simulink model "RIN251129_16_18_L2"  (R2016b)
settings: Solver=VariableStepAuto  StartTime=0.0  StopTime=0.01  RelTol=1e-3
libraries: powerlib x31, powerlib_meascontrol x13
settings Model: Creator=ADMINISTRATOR  LastModifiedBy=Victor

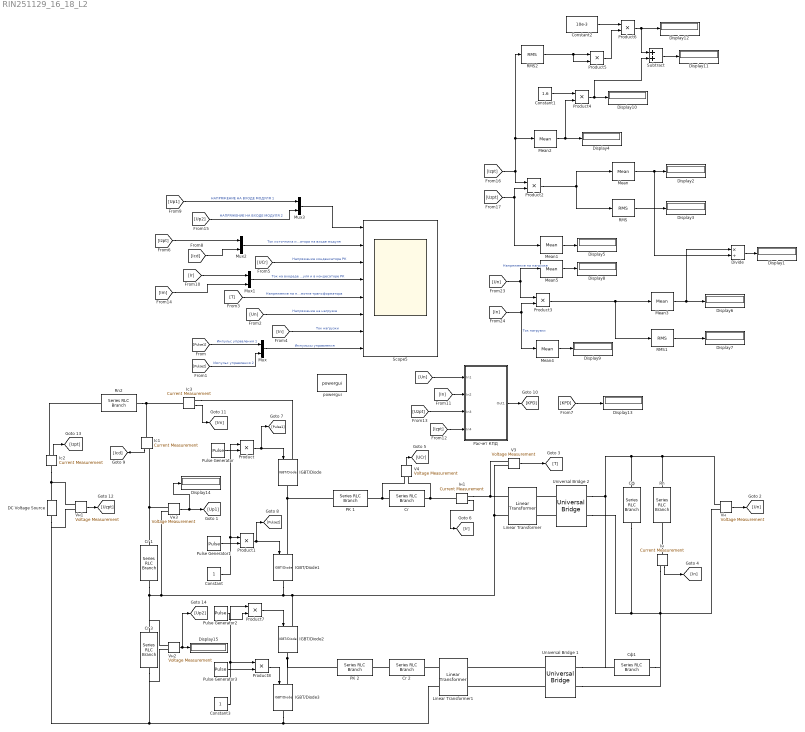
== system RIN251129_16_18_L2 ==
  " Rn" : powerlib/Elements/Series RLC Branch  LConnTagsString=__new0  RConnTagsString=__new0  BranchType=R  Resistance=4  Inductance=1e-3  SetiL0=off  InitialCurrent=0  Capacitance=1e-6  Setx0=off  InitialVoltage=0  Measurements=Branch voltage and current
  " Rn2" : powerlib/Elements/Series RLC Branch  LConnTagsString=__new0  RConnTagsString=__new0  BranchType=R  Resistance=0.3  Inductance=1e-3  SetiL0=off  InitialCurrent=0  Capacitance=1e-6  Setx0=off  InitialVoltage=0  Measurements=Branch voltage and current
  Constant : Constant
  Constant1 : Constant  Value=1.6
  Constant2 : Constant  Value=10e-3
  Constant3 : Constant
  "Cr " : powerlib/Elements/Series RLC Branch  LConnTagsString=__new0  RConnTagsString=__new0  BranchType=C  Resistance=0.001  Inductance=5e-6  SetiL0=off  InitialCurrent=0  Capacitance=1.6e-6  Setx0=off  InitialVoltage=0  Measurements=Branch voltage and current
  Cr 1 : powerlib/Elements/Series RLC Branch  LConnTagsString=__new0  RConnTagsString=__new0  BranchType=C  Resistance=0.001  Inductance=5e-6  SetiL0=off  InitialCurrent=0  Capacitance=20e-6  Setx0=off  InitialVoltage=0  Measurements=Branch voltage and current
  Cr 2 : powerlib/Elements/Series RLC Branch  LConnTagsString=__new0  RConnTagsString=__new0  BranchType=C  Resistance=0.001  Inductance=5e-6  SetiL0=off  InitialCurrent=0  Capacitance=1.6e-6  Setx0=off  InitialVoltage=0  Measurements=Branch voltage and current
  Cr 3 : powerlib/Elements/Series RLC Branch  LConnTagsString=__new0  RConnTagsString=__new0  BranchType=C  Resistance=0.001  Inductance=5e-6  SetiL0=off  InitialCurrent=0  Capacitance=20e-6  Setx0=off  InitialVoltage=0  Measurements=Branch voltage and current
  DC Voltage Source : powerlib/Electrical Sources/DC Voltage Source  Amplitude=1000  Measurements=None
  Display{1..15} (15 alike) : Display
  Divide : Product  Inputs=*/
  IGBT/Diode{,1..3} (4 alike) : powerlib/Power Electronics/IGBT//Diode  Ron=4.5e-6  Rs=1e5  Cs=inf  Measurements=off
  Ic1 : powerlib/Measurements/Current Measurement  PhasorSimulation=off  OutputType=Complex  PSBequivalent=0
  Ic2 : powerlib/Measurements/Current Measurement  PhasorSimulation=off  OutputType=Complex  PSBequivalent=0
  Ic3 : powerlib/Measurements/Current Measurement  PhasorSimulation=off  OutputType=Complex  PSBequivalent=0
  Iн : powerlib/Measurements/Current Measurement  PhasorSimulation=off  OutputType=Complex  PSBequivalent=0
  Iн1 : powerlib/Measurements/Current Measurement  PhasorSimulation=off  OutputType=Complex  PSBequivalent=0
  Linear Transformer : powerlib/Elements/Linear Transformer  UNITS=pu  NominalPower=[ 2e3 7e4 ]  winding1=[250 1e-4 1e-7]  winding2=[325 1e-4 1e-7]  ThreeWindings=off  winding3=[3.15e+05 0.7938 0.084225]  RmLm=[1e4 1e4]  Measurements=None  DataType=off
  Linear Transformer1 : powerlib/Elements/Linear Transformer  UNITS=pu  NominalPower=[ 2e3 7e4 ]  winding1=[250 1e-4 1e-7]  winding2=[325 1e-4 1e-7]  ThreeWindings=off  winding3=[3.15e+05 0.7938 0.084225]  RmLm=[1e4 1e4]  Measurements=None  DataType=off
  Mean{,1..5} (6 alike) : powerlib_meascontrol/Measurements/Mean  Freq=16e3  Vinit=0  Ts=0
  Mux{,1..3} (4 alike) : Mux  Inputs=2
  Product{,1..8} (9 alike) : Product
  Pulse Generator : DiscretePulseGenerator  PulseType=Time based  Amplitude=20  Period=1/16e3  PulseWidth=27
  Pulse Generator1 : DiscretePulseGenerator  PulseType=Time based  Amplitude=20  Period=1/16e3  PulseWidth=27  PhaseDelay=1/32e3
  Pulse Generator2 : DiscretePulseGenerator  PulseType=Time based  Amplitude=20  Period=1/18e3  PulseWidth=27  PhaseDelay=1/72e3
  Pulse Generator3 : DiscretePulseGenerator  PulseType=Time based  Amplitude=20  Period=1/18e3  PulseWidth=27  PhaseDelay=3/72e3
  RMS : powerlib_meascontrol/Measurements/RMS  TrueRMS=on  Freq=16e3  RMSInit=0  Ts=0
  RMS1 : powerlib_meascontrol/Measurements/RMS  TrueRMS=on  Freq=16e3  RMSInit=0  Ts=0
  RMS2 : powerlib_meascontrol/Measurements/RMS  TrueRMS=on  Freq=16e3  RMSInit=0  Ts=0
  Scope5 : Scope  NumInputPorts=8
  Subtract : Sum
  Universal Bridge 1 : powerlib/Power Electronics/Universal Bridge  Arms=2  SnubberResistance=1000000  SnubberCapacitance=1e-12  Device=Diodes  Ron=1e-6  Lon=0  ForwardVoltages="[  0  0  ]"  ForwardVoltage=0  GTOparameters=[ 10e-6 , 20e-6 ]  IGBTparameters=[ 1e-6 , 2e-6 ]  Measurements=None  Measurements_2=None  converterType=Rectifier
  Universal Bridge 2 : powerlib/Power Electronics/Universal Bridge  Arms=2  SnubberResistance=1000000  SnubberCapacitance=1e-12  Device=Diodes  Ron=1e-6  Lon=0  ForwardVoltages="[  0  0  ]"  ForwardVoltage=0  GTOparameters=[ 10e-6 , 20e-6 ]  IGBTparameters=[ 1e-6 , 2e-6 ]  Measurements=None  Measurements_2=None  converterType=Rectifier
  V3 : powerlib/Measurements/Voltage Measurement  PhasorSimulation=off  OutputType=Complex  PSBequivalent=0
  V4 : powerlib/Measurements/Voltage Measurement  PhasorSimulation=off  OutputType=Complex  PSBequivalent=0
  Vн{,1..3} (4 alike) : powerlib/Measurements/Voltage Measurement  PhasorSimulation=off  OutputType=Complex  PSBequivalent=0
  powergui : powerlib/powergui  Priority=1  SimulationMode=Discrete  SolverType=Tustin/Backward Euler (TBE)  SampleTime=1e-6  frequency=60  SPID=off  DisableSnubberDevices=off  DisableRonSwitches=off  DisableVfSwitches=off  SwTol=0  DisplayEquations=off  Interpol=off  ExternalGateDelay=off  methode=off  Ts=10  FunctionMessages=off  echomessages=off  HookPort=off  EnableUseOfTLC=off  x0status=blocks  frequencyindice=0  Pbase=100e6  ErrMax=1e-4  Iterations=50  UnitsV=kV  UnitsW=MW  buscounter=0  RestoreLinks=warning  ResistiveCurrentMeasurement=off  Frange=[0:2:500]  Ylog=off  Xlog=on  ShowGrid=off  save=off  variable=ZData  structure=0  ZoomFFT=off  StartTime=0.0  cycles=1  DisplayStyle=1  fundamental=60  FreqAxis=off  MaxFrequency=1000  frequencyindicesteady=1  RmsSteady=1  display=off
  РК 1 : powerlib/Elements/Series RLC Branch  LConnTagsString=__new0  RConnTagsString=__new0  BranchType=RL  Resistance=0.000001  Inductance=13.6e-6  SetiL0=off  InitialCurrent=0  Capacitance=3e-6  Setx0=off  InitialVoltage=0  Measurements=None
  РК 2 : powerlib/Elements/Series RLC Branch  LConnTagsString=__new0  RConnTagsString=__new0  BranchType=RL  Resistance=0.000001  Inductance=13.6e-6  SetiL0=off  InitialCurrent=0  Capacitance=3e-6  Setx0=off  InitialVoltage=0  Measurements=None
  Расчет КПД : Subsystem
  Сф : powerlib/Elements/Series RLC Branch  LConnTagsString=__new0  RConnTagsString=__new0  BranchType=C  Resistance=0.001  Inductance=5e-6  SetiL0=off  InitialCurrent=0  Capacitance=60e-6  Setx0=off  InitialVoltage=300  Measurements=Branch voltage and current
  Сф1 : powerlib/Elements/Series RLC Branch  LConnTagsString=__new0  RConnTagsString=__new0  BranchType=C  Resistance=0.001  Inductance=5e-6  SetiL0=off  InitialCurrent=0  Capacitance=60e-6  Setx0=off  InitialVoltage=300  Measurements=Branch voltage and current
  wires:
  Vн/1 -> [Un]
  V3/1 -> [T]
  Iн/1 -> [In]
  V4/1 -> [UCr]
  [UCr] -> Scope5/3  "Напряжение конденсатора РК"
  Iн1/1 -> [Ir]
  [In] -> Scope5/7  "Ток нагрузки"
  [Un] -> Scope5/6  "Напряжение на нагрузке"
  [T] -> Scope5/5  "Напряжение на первичной обмотке трансформатора"
  Product1/1 -> IGBT/Diode1/1, [Pulse2]
  Product/1 -> [Pulse1], IGBT/Diode/1
  [Un] -> Расчет КПД/1(In1)
  [In] -> Расчет КПД/2(In2)
  [Uzpt] -> Расчет КПД/3(In3)
  [Izpt] -> Расчет КПД/4(In4)
  Расчет КПД/1(Out1) -> [KPD]
  Pulse Generator/1 -> Product/2
  Pulse Generator1/1 -> Product1/2
  Constant/1 -> Product/1, Product1/1
  [Izpt] -> Product2/1, Mean2/1, RMS2/1
  [Uzpt] -> Product2/2, Mean1/1
  Product2/1 -> RMS/1, Mean/1
  RMS/1 -> Display3/1
  Mean1/1 -> Display5/1
  Mean2/1 -> Product4/2, Display4/1
  Product3/1 -> RMS1/1, Mean3/1
  RMS1/1 -> Display7/1
  Mean3/1 -> Divide/1, Display6/1
  Mean4/1 -> Display9/1
  Mean5/1 -> Display8/1
  [Un] -> Mean5/1, Product3/1  "Напряжение на нагрузке"
  [In] -> Product3/2, Mean4/1  "Ток нагрузки"
  Divide/1 -> Display1/1
  Mean/1 -> Divide/2, Display2/1
  Constant1/1 -> Product4/1
  RMS2/1 -> Product5/1, Product5/2
  Constant2/1 -> Product6/1
  Product5/1 -> Product6/2
  Product6/1 -> Display12/1, Subtract/1
  Product4/1 -> Subtract/2, Display10/1
  Subtract/1 -> Display11/1
  Mux2/1 -> Scope5/2  "Ток источника и конденсатора на входе модуля"
  Vн3/1 -> Display14/1, [Up1]
  [Pulse1] -> Mux/1  "Импульс управления 1"
  [Pulse2] -> Mux/2  "Импульс управления 2"
  Product8/1 -> IGBT/Diode3/1
  Product7/1 -> IGBT/Diode2/1
  Pulse Generator2/1 -> Product7/2
  Pulse Generator3/1 -> Product8/2
  Constant3/1 -> Product7/1, Product8/1
  Ic1/1 -> [Icd]
  Ic2/1 -> [Izpt]
  Ic3/1 -> [Im]
  [Ir] -> Mux1/1
  [Im] -> Mux1/2
  Mux1/1 -> Scope5/4  "Ток на входеде модуля и в кондесаторе РК"
  [Izpt] -> Mux2/1
  [Icd] -> Mux2/2
  Mux/1 -> Scope5/8  "Импульсы управления"
  Vн1/1 -> [Uzpt]
  [KPD] -> Display13/1
  Vн2/1 -> [Up2], Display15/1
  [Up2] -> Mux3/2  "НАПРЯЖЕНИЕ НА ВХОДЕ МОДУЛЯ 2"
  [Up1] -> Mux3/1  "НАПРЯЖЕНИЕ НА ВХОДЕ МОДУЛЯ 1"
  Mux3/1 -> Scope5/1
  connections:
  РК 1/LConn1 -- IGBT/Diode1/LConn1 -- IGBT/Diode/RConn1
  "Cr "/RConn1 -- V4/LConn2 -- Iн1/LConn1
  Vн/LConn1 -- Сф1/RConn1 -- Universal Bridge 1/RConn1 -- Universal Bridge 2/RConn1 -- Сф/LConn1 -- " Rn"/LConn1
  Iн/LConn1 -- " Rn"/RConn1
  V4/LConn1 -- "Cr "/LConn1 -- РК 1/RConn1
  Iн1/RConn1 -- Linear Transformer/LConn1 -- V3/LConn1
  Сф/RConn1 -- Universal Bridge 1/RConn2 -- Сф1/LConn1 -- Vн/LConn2 -- Iн/RConn1 -- Universal Bridge 2/RConn2
  Cr 1/RConn1 -- Vн2/LConn1 -- Cr 3/LConn1 -- Vн3/LConn2 -- IGBT/Diode2/LConn1 -- Linear Transformer/LConn2 -- V3/LConn2 -- IGBT/Diode1/RConn1
  Universal Bridge 2/LConn2 -- Linear Transformer/RConn2
  Universal Bridge 2/LConn1 -- Linear Transformer/RConn1
  " Rn2"/LConn1 -- Ic3/LConn1 -- Ic1/LConn1
  IGBT/Diode2/RConn1 -- IGBT/Diode3/LConn1 -- РК 2/LConn1
  Cr 2/LConn1 -- РК 2/RConn1
  Universal Bridge 1/LConn2 -- Linear Transformer1/RConn2
  Universal Bridge 1/LConn1 -- Linear Transformer1/RConn1
  Linear Transformer1/LConn1 -- Cr 2/RConn1
  Cr 1/LConn1 -- Vн3/LConn1 -- Ic1/RConn1
  Linear Transformer1/LConn2 -- Vн2/LConn2 -- Cr 3/RConn1 -- Vн1/LConn2 -- DC Voltage Source/LConn1 -- IGBT/Diode3/RConn1
  Ic2/LConn1 -- Vн1/LConn1 -- DC Voltage Source/RConn1
  Ic2/RConn1 -- " Rn2"/RConn1
  Ic3/RConn1 -- IGBT/Diode/LConn1

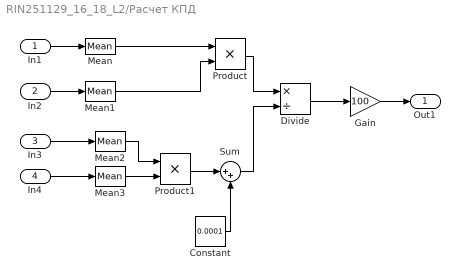
== system RIN251129_16_18_L2/Расчет КПД ==
  In1 : Inport
  In2 : Inport  Port=2
  In3 : Inport  Port=3
  In4 : Inport  Port=4
  Constant : Constant  Value=0.0001
  Divide : Product  Inputs=*/
  Gain : Gain  Gain=100
  Mean{,1..3} (4 alike) : powerlib_meascontrol/Measurements/Mean  Freq=16e3  Vinit=0  Ts=0
  Product : Product
  Product1 : Product
  Sum : Sum  Inputs=|++
  Out1 : Outport
  wires:
  Product/1 -> Divide/1
  Divide/1 -> Gain/1
  Gain/1 -> Out1/1
  In1/1 -> Mean/1
  Mean/1 -> Product/1
  In2/1 -> Mean1/1
  Mean1/1 -> Product/2
  In3/1 -> Mean2/1
  Mean2/1 -> Product1/1
  In4/1 -> Mean3/1
  Mean3/1 -> Product1/2
  Product1/1 -> Sum/1
  Sum/1 -> Divide/2
  Constant/1 -> Sum/2
